simulink model "simulink_aufg2_a"  (Simulink 7.7)
settings: Solver=ode45  StartTime=0.0  StopTime=35.0  RelTol=1e-3
settings Model: Creator=myers  LastModifiedBy=hexren

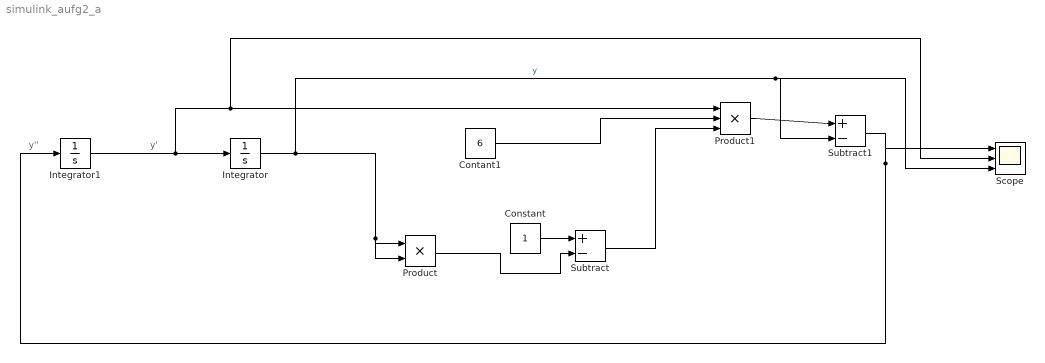
== system simulink_aufg2_a ==
  note: y'
  note: y''
  Constant : Constant
  Contant1 : Constant  Value=6
  Integrator : Integrator
  Integrator1 : Integrator  InitialCondition=1
  Product : Product  RndMeth=Zero
  Product1 : Product  Inputs=3  RndMeth=Zero
  Scope : Scope  NumInputPorts=3
      settings: YMin=-5~-5~-5  YMax=5~5~5
  Subtract : Sum  Inputs=+-
  Subtract1 : Sum  Inputs=+-
  wires:
  Integrator1/1 -> Integrator/1, Product1/1, Scope/2
  Integrator/1 -> Product/1, Product/2, Subtract1/2, Scope/3  "y"
  Constant/1 -> Subtract/1
  Product/1 -> Subtract/2
  Subtract/1 -> Product1/3
  Contant1/1 -> Product1/2
  Product1/1 -> Subtract1/1
  Subtract1/1 -> Integrator1/1, Scope/1
